simulink model "MassSpringDamperCut"  (R2025a)
settings: Solver=FixedStepDiscrete  StartTime=0.0  StopTime=3  FixedStep=0.01  RelTol=1e-3  AbsTol=1e-3  EnableMultiTasking=on
PreLoadFcn:
  | disp('Mass-spring-damper parameters:')
  | disp('m = 10');
  | disp('k = 1e3');
  | disp('b = 1e2');
  | disp('F = 10');
  | 
  | m = 10; %mass
  | k = 1e3; %stiffness
  | b = 1e2; %damping
  | F = 10; %input force
undefined symbols (not defined in the file): a79c, b1df, DiscIntNeverNeededParam, f927c76d
settings Model: Creator=guirl  LastModifiedBy=guirl
settings SolverCC: AutoScaleAbsTol=off  AlgebraicLoopSolver=TrustRegion
settings OptimizationCC: LifeSpan=inf
settings DebuggingCC: UnconnectedInputMsg=warning  UnconnectedOutputMsg=warning  UnconnectedLineMsg=warning  SFUnexpectedBacktrackingDiag=warning  SFNoUnconditionalDefaultTransitionDiag=warning  ArithmeticOperatorsInVariantConditions=warning
settings ModelReferenceCC: EnableRefExpFcnMdlSchedulingChecks=on
settings SFSimCC: SimUseLocalCustomCode=off  CustomCodeUndefinedFunction=UseInterfaceOnly
settings RTWCC: RTWUseLocalCustomCode=off  GPUComputeCapability=3.5  DLArmComputeVersion=19.05
settings CodeAppCC: StateflowObjectComments=on
settings GRTTargetCC: TargetLangStandard=C89/C90 (ANSI)
settings ConfigComp: CovMetricSettings=dw  CovSaveCumulativeToWorkspaceVar=on  CovSaveSingleToWorkspaceVar=on  CovExternalEMLEnable=off
settings SimscapeCC: SimscapeNormalizeSystem=off  SimscapeLogType=all  SimscapeLogSimulationStatistics=on  SimscapeLogLimitData=off

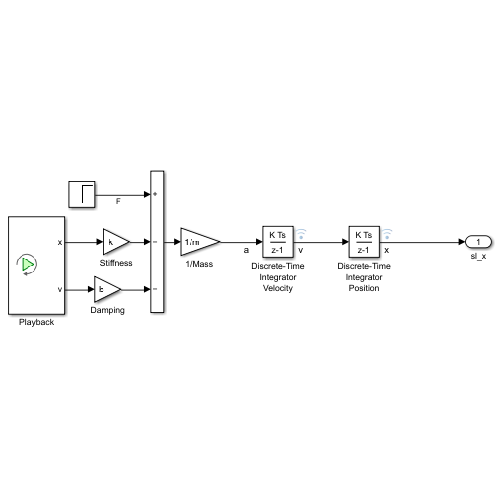
[thumbnail: Simulink's stored preview of the top-level diagram]
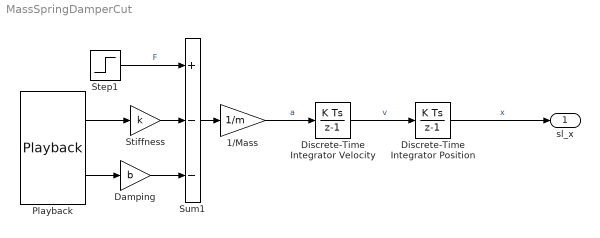
== system MassSpringDamperCut ==
  "1/Mass " : Gain  Gain=1/m  SaturateOnIntegerOverflow=on  OutDataTypeStr=Inherit: Same as input  ParamDataTypeStr=Inherit: Same as input
  Damping : Gain  Gain=b  SaturateOnIntegerOverflow=on  OutDataTypeStr=Inherit: Same as input  ParamDataTypeStr=Inherit: Same as input
  Discrete-Time Integrator Position : DiscreteIntegrator  SampleTime=-1  ICPrevOutput=DiscIntNeverNeededParam  ICPrevScaledInput=DiscIntNeverNeededParam
  Discrete-Time Integrator Velocity : DiscreteIntegrator  SampleTime=-1  ICPrevOutput=DiscIntNeverNeededParam  ICPrevScaledInput=DiscIntNeverNeededParam
  Playback : Playback  NumPorts=2  PartName=f927c76d-a79c-49fc-b1df-3f19e39651cb  TableView=on  TablePosition=Bottom
  Step1 : Step  After=F  SampleTime=0.01
  Stiffness : Gain  Gain=k  SaturateOnIntegerOverflow=on  OutDataTypeStr=Inherit: Same as input  ParamDataTypeStr=Inherit: Same as input
  Sum1 : Sum  Inputs=+--  InputSameDT=on  SaturateOnIntegerOverflow=on  OutDataTypeStr=Inherit: Same as first input
  sl_x : Outport
  wires:
  "1/Mass "/1 -> Discrete-Time Integrator Velocity/1  "a"
  Sum1/1 -> "1/Mass "/1
  Discrete-Time Integrator Position/1 -> sl_x/1  "x"
  Discrete-Time Integrator Velocity/1 -> Discrete-Time Integrator Position/1  "v"
  Step1/1 -> Sum1/1  "F"
  Damping/1 -> Sum1/3
  Stiffness/1 -> Sum1/2
  Playback/1 -> Stiffness/1
  Playback/2 -> Damping/1
